simulink model "example2"  (Simulink 4.00)
settings: Solver=ode45  StartTime=0.0  StopTime=20.0  MaxStep=0.02  RelTol=1e-3
values from neighbouring files (symbols this model uses):
  A = [0  1; 0  -1]    [params.mat]
  Ae = [-9  1; -41  -1]    [params.mat]
  B = [0 1]    [params.mat]
  C = [2 0]    [params.mat]
  G = [4.5 20.5]    [params.mat]
  K = [1 1]    [params.mat]
  M = [22.0625 284.125]    [params.mat]
  N = 33.0625    [params.mat]
libraries: simulink3 x2
settings Model: LastModifiedBy=gordon

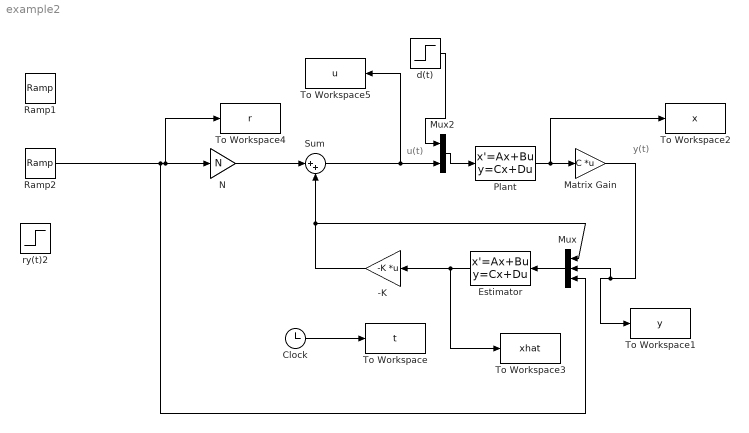
== system example2 ==
  note: u(t)
  note: y(t)
  -K : Gain  Orientation=left  Gain=-K  Multiplication=Matrix(K*u)  SaturateOnIntegerOverflow=on
  Clock : Clock
      settings: DisplayTime=off  Decimation=10
  Estimator : StateSpace  Orientation=left  A=Ae  B=[B G M]  C=[1 0;0 1]  D=[0 0 0;0 0 0]  X0=0  AbsoluteTolerance=auto  Realization=auto
  Matrix Gain : Gain  Gain=C  Multiplication=Matrix(K*u)  SaturateOnIntegerOverflow=on
  Mux : Mux  Orientation=left  Inputs=3
  Mux2 : Mux  Inputs=2
  N : Gain  Gain=N  Multiplication=Element-wise(K.*u)  SaturateOnIntegerOverflow=on
  Plant : StateSpace  A=A  B=[E B]  C=[1 0;0 1]  D=[0 0; 0 0]  X0=0  AbsoluteTolerance=auto  Realization=auto
  Ramp1 : simulink3/Sources/Ramp  slope=1  start=0  X0=0
  Ramp2 : simulink3/Sources/Ramp  slope=1  start=0  X0=0
  Sum : Sum  Inputs=|++  SaturateOnIntegerOverflow=on
  To Workspace : ToWorkspace  VariableName=t  SampleTime=-1  SaveFormat=Array
  To Workspace1 : ToWorkspace  VariableName=y  SampleTime=-1  SaveFormat=Array
  To Workspace2 : ToWorkspace  VariableName=x  SampleTime=-1  SaveFormat=Array
  To Workspace3 : ToWorkspace  VariableName=xhat  SampleTime=-1  SaveFormat=Array
  To Workspace4 : ToWorkspace  VariableName=r  SampleTime=-1  SaveFormat=Array
  To Workspace5 : ToWorkspace  VariableName=u  SampleTime=-1  SaveFormat=Array
  d(t) : Step  Time=10  Before=0  After=0  SampleTime=0
  ry(t)2 : Step  Time=1  Before=0  After=1  SampleTime=0
  wires:
  Mux/1 -> Estimator/1
  Sum/1 -> To Workspace5/1, Mux2/2
  Ramp2/1 -> N/1, To Workspace4/1, Mux/3
  N/1 -> Sum/1
  Plant/1 -> Matrix Gain/1, To Workspace2/1
  Matrix Gain/1 -> To Workspace1/1, Mux/2
  Clock/1 -> To Workspace/1
  Mux2/1 -> Plant/1
  d(t)/1 -> Mux2/1
  Estimator/1 -> To Workspace3/1, -K/1
  -K/1 -> Sum/2, Mux/1
